simulink model "EMPlanner_cs2018"  (R2018a)
settings: Solver=ode5  StartTime=0.0  StopTime=120  FixedStep=1/1000  RelTol=1e-3
PreLoadFcn:
  | mbxruntime.callbacks.PreLoadFcn(bdroot);
PostLoadFcn:
  | mbxruntime.callbacks.PostLoadFcn(bdroot);
InitFcn:
  | mbxruntime.callbacks.InitFcn(bdroot);
StartFcn:
  | mbxruntime.callbacks.StartFcn(bdroot);
StopFcn:
  | mbxruntime.callbacks.StopFcn(bdroot);
model workspace (MAT data in the model file):
  mbox_table : struct (value not decoded)
  model_closed = 0
  sim_status = 0
undefined symbols (not defined in the file or in its folder): aubr, c_factor, cf, cr, DiscIntNeverNeededParam, global_path_x, global_path_y, KD_PID_distance, KD_PID_speed, KI_PID_distance, KI_PID_speed, KP_PID_distance, KP_PID_speed, la, lb, LQR_K1, LQR_K2, LQR_K3, LQR_K4, m, rack_displacement, right_wheel_ground, tablebr, vubr, vx_break_point, warningInitialVelocity, x0
libraries: PreScanSimulinkLibrary x21, simulink x19, simulink_extras x6, Solver_SF x1
(part 8 of 9)

== matlab function EMPlanner_cs2018/Audi_A8_Sedan_1/decision&planning module1/referenceline provider/MATLAB Function5 ==
  data: x_set input; match_point_index_set output; y_set input; frenet_path_x input; frenet_path_y input; frenet_path_heading input; frenet_path_kappa input; proj_x_set output; proj_y_set output; proj_heading_set output; proj_kappa_set output
function [match_point_index_set,proj_x_set,proj_y_set,proj_heading_set,proj_kappa_set] = ...
    fcn(x_set,y_set,frenet_path_x,frenet_path_y,frenet_path_heading,frenet_path_kappa)
%该函数将批量计算x_set，y_set中的xy，在frenet_path下的投影的信息
%输入 x_set,y_set，待投影的点的集合
%x_set,y_set,frenet_path_x,frenet_path_y,frenet_path_heading,frenet_path_kappa
%曲线在直角坐标系下的x，y，heading，kappa
%输出：match_point_index_set 匹配点在frenet_path下的编号的集合(即从全局路径第一个点开始数，第几个点是匹配点)
%     proj_x y heading kappa 投影的x,y,heading,kappa的集合

% 由于事先不知道x_set中到底有多少个点需要投影，因此事先声明一个最大的数量的点作为缓冲
n = 128;
% 并且由于不知道投影点的个数，所以也不知道输出的个数，因此输出也要做缓冲，用nan表示不存在的点
% 输出最多输出128个
% 输出初始化
match_point_index_set = ones(n,1) * nan;
proj_x_set = ones(n,1) * nan;
proj_y_set = ones(n,1) * nan;
proj_heading_set = ones(n,1) * nan;
proj_kappa_set = ones(n,1) * nan;

%找匹配点，需要利用上一个周期的结果作为下一个周期遍历的起点，因此需要声明两个全局变量
persistent is_first_run;
persistent pre_match_point_index_set;
persistent pre_frenet_path_x;
persistent pre_frenet_path_y;
persistent pre_frenet_path_heading;
persistent pre_frenet_path_kappa;
%算法主函数入口

if isempty(is_first_run)
    %该if分支表示函数首次运行
    is_first_run = 0;
    pre_frenet_path_x = frenet_path_x;
    pre_frenet_path_y = frenet_path_y;
    pre_frenet_path_heading = frenet_path_heading;
    pre_frenet_path_kappa = frenet_path_kappa;
    %要记录首次运行计算的匹配点的结果供下个周期运行，先初始化
    pre_match_point_index_set = ones(n,1) * nan;
    %对x_set,y_set的点做遍历，找到他们的匹配点
    for i = 1 : length(x_set)
        %首次运行时，没有任何提示，只能从frenet path的第一个点开始找
        if isnan(x_set(i))
            break;
        end
        start_search_index = 1;
        % 声明increase_count，用于表示在遍历时distance连续增加的个数
        increase_count = 0;
        % 开始遍历
        min_distance = inf;
        for j = start_search_index : length(frenet_path_x)
            distance = (x_set(i) - frenet_path_x(j))^2 + (y_set(i) - frenet_path_y(j))^2;
            if distance < min_distance
                min_distance = distance;
                match_point_index_set(i) = j;
                increase_count = 0;
            else
                increase_count = increase_count + 1;
            end
            %如果distance连续增加50次就不要再遍历了，节省时间
            if increase_count > 50
                break;
            end
        end
        
        %如何通过匹配点计算投影点，请参见《自动驾驶控制算法第七讲》
        %或《自动驾驶决策规划算法》第一章第三节
        
        %取出匹配点的编号
        match_point_index = match_point_index_set(i);
        %取出匹配点的信息
        match_point_x = frenet_path_x(match_point_index);
        match_point_y = frenet_path_y(match_point_index);
        match_point_heading = frenet_path_heading(match_point_index);
        match_point_kappa = frenet_path_kappa(match_point_index);
        %计算匹配点的方向向量与法向量
        vector_match_point = [match_point_x;match_point_y];
        vector_match_point_direction = [cos(match_point_heading);sin(match_point_heading)];
        %声明待投影点的位矢
        vector_r = [x_set(i);y_set(i)];
        
       %通过匹配点计算投影点
       vector_d = vector_r - vector_match_point;
       ds = vector_d' * vector_match_point_direction;
       vector_proj_point = vector_match_point + ds * vector_match_point_direction;
       proj_heading = match_point_heading + match_point_kappa * ds;
       proj_kappa = match_point_kappa;
       %计算结果输出
       proj_x_set(i) = vector_proj_point(1);
       proj_y_set(i) = vector_proj_point(2);
       proj_heading_set(i) = proj_heading;
       proj_kappa_set(i) = proj_kappa;
    end
    %匹配点的计算结果保存，供下一个周期使用
    pre_match_point_index_set = match_point_index_set;
else
    %此if分支表示不是首次运行
    
    %对每个x_set上的点做处理
    for i = 1 : length(x_set)
        %不是首次运行，对于点x_set(i),y_set(i)来说,start_search_index =
        %pre_match_point_index_set(i)
        start_search_index = pre_match_point_index_set(i);%上个周期匹配点的编号作为本周期搜索的起点
        %%%%%%%%%%%%
        increase_count_limit = 5;
        if isnan(start_search_index)
            increase_count_limit = 50;
            start_search_index = 1;
        end
        %%%%%%%%%%%%%%
        % 声明increase_count，用于表示在遍历时distance连续增加的个数
        increase_count = 0;
        % 开始遍历
        %这里多一个步骤，判断遍历的方向
        %计算上个周期匹配点的位矢
        vector_pre_match_point = [pre_frenet_path_x(start_search_index);pre_frenet_path_y(start_search_index)];
        vector_pre_match_point_direction = ...
            [cos(pre_frenet_path_heading(start_search_index));sin(pre_frenet_path_heading(start_search_index))];
        %判断遍历的方向
        flag = ([x_set(i);y_set(i)] - vector_pre_match_point)' * vector_pre_match_point_direction;
        min_distance = inf;
        if flag > 0.001
            for j = start_search_index : length(frenet_path_x)
                distance = (x_set(i) - frenet_path_x(j))^2 + (y_set(i) - frenet_path_y(j))^2;
                if distance < min_distance
                    min_distance = distance;
                    match_point_index_set(i) = j;
                    increase_count = 0;
                else
                    increase_count = increase_count + 1;
                end
                %如果distance连续增加5次就不要再遍历了，节省时间
                if increase_count > 5
                    break;
                end
            end
        elseif flag < - 0.001
            for j = start_search_index : -1 : 1
                distance = (x_set(i) - frenet_path_x(j))^2 + (y_set(i) - frenet_path_y(j))^2;
                if distance < min_distance
                    min_distance = distance;
                    match_point_index_set(i) = j;
                    increase_count = 0;
                else
                    increase_count = increase_count + 1;
                end
                %如果distance连续增加5次就不要再遍历了，节省时间
                if increase_count > increase_count_limit
                    break;
                end
            end
        else
            match_point_index_set(i) = start_search_index;
        end
        
        %如何通过匹配点计算投影点，请参见《自动驾驶控制算法第七讲》
        %或《自动驾驶决策规划算法》第一章第三节
        
        %取出匹配点的编号
        match_point_index = match_point_index_set(i);
        %取出匹配点的信息
        match_point_x = frenet_path_x(match_point_index);
        match_point_y = frenet_path_y(match_point_index);
        match_point_heading = frenet_path_heading(match_point_index);
        match_point_kappa = frenet_path_kappa(match_point_index);
        %计算匹配点的方向向量与法向量
        vector_match_point = [match_point_x;match_point_y];
        vector_match_point_direction = [cos(match_point_heading);sin(match_point_heading)];
        %声明待投影点的位矢
        vector_r = [x_set(i);y_set(i)];
        
       %通过匹配点计算投影点
       vector_d = vector_r - vector_match_point;
       ds = vector_d' * vector_match_point_direction;
       vector_proj_point = vector_match_point + ds * vector_match_point_direction;
       proj_heading = match_point_heading + match_point_kappa * ds;
       proj_kappa = match_point_kappa;
       %计算结果输出
       proj_x_set(i) = vector_proj_point(1);
       proj_y_set(i) = vector_proj_point(2);
       proj_heading_set(i) = proj_heading;
       proj_kappa_set(i) = proj_kappa;
  
    end
    %匹配点的计算结果保存，供下一个周期使用
    pre_match_point_index_set = match_point_index_set;
    pre_frenet_path_x = frenet_path_x;
    pre_frenet_path_y = frenet_path_y;
    pre_frenet_path_heading = frenet_path_heading;
    pre_frenet_path_kappa = frenet_path_kappa;
end

== matlab function EMPlanner_cs2018/Audi_A8_Sedan_1/perception module/data handle and transfer ==
  data: range input; obs_x_set_global output; theta input; velocity input; velocity_heading input; host_x input; host_y input; host_heading input; obs_y_set_global output; obs_velocity_set_global output; obs_heading_set_global output
function [obs_x_set_global,obs_y_set_global,obs_velocity_set_global,obs_heading_set_global] = fcn(range,theta,velocity,velocity_heading,host_x,host_y,host_heading)
%%%数据处理与坐标转换
obs_x_set_global = ones(32,1) * nan ;
obs_y_set_global = ones(32,1) * nan;
obs_velocity_set_global = ones(32,1) * nan;
obs_heading_set_global = ones(32,1) * nan;
theta_transfer = -1 * theta * pi / 180;
heading_transfer = (-velocity_heading + ones(32,1)*90) * pi / 180 ;
x_transfer = range .* cos(theta_transfer + host_heading);
y_transfer = range .* sin(theta_transfer + host_heading);
for i = 1:32
    if range(i) ~= 0
        obs_x_set_global(i) = x_transfer(i) + host_x + 2.16*cos(host_heading);
        obs_y_set_global(i) = y_transfer(i) + host_y + 2.16*sin(host_heading);
        obs_heading_set_global(i) = heading_transfer(i);
        obs_velocity_set_global(i) = velocity(i);
    end
end

== matlab function EMPlanner_cs2018/Audi_A8_Sedan_2/PathFollower_Preview_1/LateralController/Calculate delta steering error/eml_delta_steering_error ==
  data: v_x_vehicle input; v_x_vehicle_Min input; t_Preview_LatCtrl input; delta_steeringwheeltotal output; v_y_vehicle input; yawrate_vehicle input; CorneringStiffness_Tyres_Front input; CorneringStiffness_Tyres_Rear input; m_vehicle_total input; inertia_z_vehicle_total input; e_Lat input size=10; Pos_x_CoG_Vehicle input; wheelbase input; RefreshCounter parameter
function delta_steeringwheeltotal = eml_delta_steering_error(v_x_vehicle,v_x_vehicle_Min,t_Preview_LatCtrl,v_y_vehicle,yawrate_vehicle,CorneringStiffness_Tyres_Front,CorneringStiffness_Tyres_Rear,m_vehicle_total,inertia_z_vehicle_total,e_Lat,Pos_x_CoG_Vehicle,wheelbase,RefreshCounter)

delta_steeringwheeltotal = emlfcn_delta_steering_error(v_x_vehicle,v_x_vehicle_Min,t_Preview_LatCtrl,v_y_vehicle,yawrate_vehicle,CorneringStiffness_Tyres_Front,CorneringStiffness_Tyres_Rear,m_vehicle_total,inertia_z_vehicle_total,e_Lat,Pos_x_CoG_Vehicle,wheelbase,RefreshCounter);

% end function

== matlab function EMPlanner_cs2018/Audi_A8_Sedan_1/decision&planning module1/EM Planner/MATLAB Function7 ==
  data: s input; trajectory_x output; s_dot input; s_dot2 input; relative_time input; current_time input; path_s input; trajectory_x_init input; trajectory_y_init input; trajectory_heading_init input; trajectory_kappa_init input; trajectory_y output; trajectory_heading output; trajectory_kappa output; trajectory_speed output; trajectory_accel output; trajectory_time output
function [trajectory_x,trajectory_y,trajectory_heading,trajectory_kappa,trajectory_speed,trajectory_accel,trajectory_time] = ...
    fcn(s,s_dot,s_dot2,relative_time,current_time,path_s,trajectory_x_init,trajectory_y_init,trajectory_heading_init,trajectory_kappa_init)

n = 401;
trajectory_x = zeros(n,1);
trajectory_y = zeros(n,1);
trajectory_heading = zeros(n,1);
trajectory_kappa = zeros(n,1);
trajectory_speed = zeros(n,1);

trajectory_accel = zeros(n,1);

trajectory_time = zeros(n,1);
for i = 1:n-1
    trajectory_x(i) = interp1(path_s,trajectory_x_init,s(i));
    trajectory_y(i) = interp1(path_s,trajectory_y_init,s(i));
    trajectory_heading(i) = interp1(path_s,trajectory_heading_init,s(i));
    trajectory_kappa(i) = interp1(path_s,trajectory_kappa_init,s(i));
    trajectory_time(i) = relative_time(i) + current_time;
    trajectory_speed(i) = s_dot(i);
    trajectory_accel(i) = s_dot2(i);
end
trajectory_x(end) = trajectory_x_init(end);
trajectory_y(end) = trajectory_y_init(end);
trajectory_heading(end) = trajectory_heading_init(end);
trajectory_kappa(end) = trajectory_kappa_init(end);
trajectory_time(end) = relative_time(end) + current_time;
trajectory_speed(end) = s_dot(end);
trajectory_accel(end) = s_dot2(end);

== matlab function EMPlanner_cs2018/Audi_A8_Sedan_1/decision&planning module1/EM Planner/path decision and planning/generate obs SL/MATLAB Function5 ==
  data: x_set input; match_point_index_set output; y_set input; frenet_path_x input; frenet_path_y input; frenet_path_heading input; frenet_path_kappa input; proj_x_set output; proj_y_set output; proj_heading_set output; proj_kappa_set output
function [match_point_index_set,proj_x_set,proj_y_set,proj_heading_set,proj_kappa_set] = ...
    fcn(x_set,y_set,frenet_path_x,frenet_path_y,frenet_path_heading,frenet_path_kappa)
%该函数将批量计算x_set，y_set中的xy，在frenet_path下的投影的信息
%输入 x_set,y_set，待投影的点的集合
%x_set,y_set,frenet_path_x,frenet_path_y,frenet_path_heading,frenet_path_kappa
%曲线在直角坐标系下的x，y，heading，kappa
%输出：match_point_index_set 匹配点在frenet_path下的编号的集合(即从全局路径第一个点开始数，第几个点是匹配点)
%     proj_x y heading kappa 投影的x,y,heading,kappa的集合

% 由于事先不知道x_set中到底有多少个点需要投影，因此事先声明一个最大的数量的点作为缓冲
n = 128;
% 并且由于不知道投影点的个数，所以也不知道输出的个数，因此输出也要做缓冲，用nan表示不存在的点
% 输出最多输出128个
% 输出初始化
match_point_index_set = ones(n,1) * nan;
proj_x_set = ones(n,1) * nan;
proj_y_set = ones(n,1) * nan;
proj_heading_set = ones(n,1) * nan;
proj_kappa_set = ones(n,1) * nan;

%找匹配点，需要利用上一个周期的结果作为下一个周期遍历的起点，因此需要声明两个全局变量
persistent is_first_run;
persistent pre_match_point_index_set;
persistent pre_frenet_path_x;
persistent pre_frenet_path_y;
persistent pre_frenet_path_heading;
persistent pre_frenet_path_kappa;
%算法主函数入口

if isempty(is_first_run)
    %该if分支表示函数首次运行
    is_first_run = 0;
    pre_frenet_path_x = frenet_path_x;
    pre_frenet_path_y = frenet_path_y;
    pre_frenet_path_heading = frenet_path_heading;
    pre_frenet_path_kappa = frenet_path_kappa;
    %要记录首次运行计算的匹配点的结果供下个周期运行，先初始化
    pre_match_point_index_set = ones(n,1) * nan;
    %对x_set,y_set的点做遍历，找到他们的匹配点
    for i = 1 : length(x_set)
        if isnan(x_set(i))
            break;
        end
        %首次运行时，没有任何提示，只能从frenet path的第一个点开始找
        start_search_index = 1;
        % 声明increase_count，用于表示在遍历时distance连续增加的个数
        increase_count = 0;
        % 开始遍历
        min_distance = inf;
        for j = start_search_index : length(frenet_path_x)
            distance = (x_set(i) - frenet_path_x(j))^2 + (y_set(i) - frenet_path_y(j))^2;
            if distance < min_distance
                min_distance = distance;
                match_point_index_set(i) = j;
                increase_count = 0;
            else
                increase_count = increase_count + 1;
            end
            %如果distance连续增加50次就不要再遍历了，节省时间
            if increase_count > 50
                break;
            end
        end
        
        %如何通过匹配点计算投影点，请参见《自动驾驶控制算法第七讲》
        %或《自动驾驶决策规划算法》第一章第三节
        
        %取出匹配点的编号
        match_point_index = match_point_index_set(i);
        %取出匹配点的信息
        match_point_x = frenet_path_x(match_point_index);
        match_point_y = frenet_path_y(match_point_index);
        match_point_heading = frenet_path_heading(match_point_index);
        match_point_kappa = frenet_path_kappa(match_point_index);
        %计算匹配点的方向向量与法向量
        vector_match_point = [match_point_x;match_point_y];
        vector_match_point_direction = [cos(match_point_heading);sin(match_point_heading)];
        %声明待投影点的位矢
        vector_r = [x_set(i);y_set(i)];
        
       %通过匹配点计算投影点
       vector_d = vector_r - vector_match_point;
       ds = vector_d' * vector_match_point_direction;
       vector_proj_point = vector_match_point + ds * vector_match_point_direction;
       proj_heading = match_point_heading + match_point_kappa * ds;
       proj_kappa = match_point_kappa;
       %计算结果输出
       proj_x_set(i) = vector_proj_point(1);
       proj_y_set(i) = vector_proj_point(2);
       proj_heading_set(i) = proj_heading;
       proj_kappa_set(i) = proj_kappa;
    end
    %匹配点的计算结果保存，供下一个周期使用
    pre_match_point_index_set = match_point_index_set;
else
    %此if分支表示不是首次运行
    
    %对每个x_set上的点做处理
    for i = 1 : length(x_set)
        %不是首次运行，对于点x_set(i),y_set(i)来说,start_search_index =
        %pre_match_point_index_set(i)
        start_search_index = pre_match_point_index_set(i);%上个周期匹配点的编号作为本周期搜索的起点
        %%%%%%%%%%%%
        increase_count_limit = 5;
        if isnan(start_search_index)
            increase_count_limit = 50;
            start_search_index = 1;
        end
        %%%%%%%%%%%%%%
        % 声明increase_count，用于表示在遍历时distance连续增加的个数
        increase_count = 0;
        % 开始遍历
        %这里多一个步骤，判断遍历的方向
        %计算上个周期匹配点的位矢
        vector_pre_match_point = [pre_frenet_path_x(start_search_index);pre_frenet_path_y(start_search_index)];
        vector_pre_match_point_direction = ...
            [cos(pre_frenet_path_heading(start_search_index));sin(pre_frenet_path_heading(start_search_index))];
        %判断遍历的方向
        flag = ([x_set(i);y_set(i)] - vector_pre_match_point)' * vector_pre_match_point_direction;
        min_distance = inf;
        if flag > 0.001
            for j = start_search_index : length(frenet_path_x)
                distance = (x_set(i) - frenet_path_x(j))^2 + (y_set(i) - frenet_path_y(j))^2;
                if distance < min_distance
                    min_distance = distance;
                    match_point_index_set(i) = j;
                    increase_count = 0;
                else
                    increase_count = increase_count + 1;
                end
                %如果distance连续增加5次就不要再遍历了，节省时间
                if increase_count > 5
                    break;
                end
            end
        elseif flag < - 0.001
            for j = start_search_index : -1 : 1
                distance = (x_set(i) - frenet_path_x(j))^2 + (y_set(i) - frenet_path_y(j))^2;
                if distance < min_distance
                    min_distance = distance;
                    match_point_index_set(i) = j;
                    increase_count = 0;
                else
                    increase_count = increase_count + 1;
                end
                %如果distance连续增加5次就不要再遍历了，节省时间
                if increase_count > increase_count_limit
                    break;
                end
            end
        else
            match_point_index_set(i) = start_search_index;
        end
        
        %如何通过匹配点计算投影点，请参见《自动驾驶控制算法第七讲》
        %或《自动驾驶决策规划算法》第一章第三节
        
        %取出匹配点的编号
        match_point_index = match_point_index_set(i);
        %取出匹配点的信息
        match_point_x = frenet_path_x(match_point_index);
        match_point_y = frenet_path_y(match_point_index);
        match_point_heading = frenet_path_heading(match_point_index);
        match_point_kappa = frenet_path_kappa(match_point_index);
        %计算匹配点的方向向量与法向量
        vector_match_point = [match_point_x;match_point_y];
        vector_match_point_direction = [cos(match_point_heading);sin(match_point_heading)];
        %声明待投影点的位矢
        vector_r = [x_set(i);y_set(i)];
        
       %通过匹配点计算投影点
       vector_d = vector_r - vector_match_point;
       ds = vector_d' * vector_match_point_direction;
       vector_proj_point = vector_match_point + ds * vector_match_point_direction;
       proj_heading = match_point_heading + match_point_kappa * ds;
       proj_kappa = match_point_kappa;
       %计算结果输出
       proj_x_set(i) = vector_proj_point(1);
       proj_y_set(i) = vector_proj_point(2);
       proj_heading_set(i) = proj_heading;
       proj_kappa_set(i) = proj_kappa;
  
    end
    %匹配点的计算结果保存，供下一个周期使用
    pre_match_point_index_set = match_point_index_set;
    pre_frenet_path_x = frenet_path_x;
    pre_frenet_path_y = frenet_path_y;
    pre_frenet_path_heading = frenet_path_heading;
    pre_frenet_path_kappa = frenet_path_kappa;
end

== stateflow chart EMPlanner_cs2018/Audi_A8_Sedan_1/Chart ==
  (default) -> (junction 5)
  (junction 5) -> (junction 7)
  (junction 7) -> (junction 9) [order 1] : [i >= 100]
  (junction 7) -> (junction 13) [order 2] : {
      | i = i + 1;
      | }
  (junction 9) -> (junction 11) : {
      | do_planning;
      | i = 1;
      | }
  (junction 11) -> (junction 13)
  (junction 13) -> (junction 16)
  (junction 16) -> (junction 18) [order 1] : [j >= 10]
  (junction 16) -> (junction 22) [order 2] : {
      | j = j + 1;
      | }
  (junction 18) -> (junction 20) : {
      | do_control;
      | j = 1;
      | }
  (junction 20) -> (junction 22)
  (junction 22) -> (junction 25)
  data: i local =1; j local =1; k local =1
  events: do_planning output FUNCTION_CALL_EVENT; do_control output FUNCTION_CALL_EVENT

== matlab function EMPlanner_cs2018/Audi_A8_Sedan_1/decision&planning module1/EM Planner/MATLAB Function1 ==
  data: qp_path_s input; qp_path_l input; dp_path_s input; dp_path_l input; l_lb input; l_ub input
function  fcn(qp_path_s,qp_path_l,dp_path_s,dp_path_l,l_lb,l_ub)
coder.extrinsic('plot')
plot(qp_path_s,qp_path_l,dp_path_s,dp_path_l,dp_path_s,l_lb,dp_path_s,l_ub);

== matlab function EMPlanner_cs2018/Audi_A8_Sedan_1/decision&planning module1/EM Planner/MATLAB Function8 ==
  data: trajectory_x input; trajectory_x_final output; trajectory_y input; trajectory_heading input; trajectory_kappa input; trajectory_speed input; trajectory_accel input; trajectory_time input; stitch_x input; stitch_y input; stitch_heading input; stitch_kappa input; stitch_speed input; stitch_accel input; stitch_time input; trajectory_y_final output; trajectory_heading_final output; trajectory_kappa_final output; trajectory_speed_final output; trajectory_accel_final output; trajectory_time_final output
function [trajectory_x_final,trajectory_y_final,trajectory_heading_final,trajectory_kappa_final,...
          trajectory_speed_final,trajectory_accel_final,trajectory_time_final] = fcn(trajectory_x,...
          trajectory_y,trajectory_heading,trajectory_kappa,trajectory_speed,trajectory_accel,trajectory_time,...
          stitch_x,stitch_y,stitch_heading,stitch_kappa,stitch_speed,stitch_accel,stitch_time)
n = 401 + 20;
trajectory_x_final = zeros(n,1);
trajectory_y_final = zeros(n,1);
trajectory_heading_final = zeros(n,1);
trajectory_kappa_final = zeros(n,1);
trajectory_speed_final = zeros(n,1);
trajectory_accel_final = zeros(n,1);
trajectory_time_final = zeros(n,1);

trajectory_x_final = [stitch_x;trajectory_x];
trajectory_y_final = [stitch_y;trajectory_y];
trajectory_heading_final = [stitch_heading;trajectory_heading];
trajectory_kappa_final = [stitch_kappa;trajectory_kappa];
trajectory_speed_final = [stitch_speed;trajectory_speed];
trajectory_accel_final = [stitch_accel;trajectory_accel];
trajectory_time_final = [stitch_time;trajectory_time];

== matlab function EMPlanner_cs2018/Audi_A8_Sedan_1/control module1/control main/chassic steering system/MATLAB Function ==
  data: u input; right_steer output; la input; lb input
function right_steer = fcn(u,la,lb)
if abs(u)<1e-2
   right_steer = u;
else
   R =  (la+lb)/tan(u);
   right_steer = atan((la+lb)/(R+1.624/2));
end

== matlab function EMPlanner_cs2018/Audi_A8_Sedan_1/control module1/control main/lateral control LQR/calc lqr K ==
  data: k1 input; k output; k2 input; k3 input; k4 input; vx input
function k  = fcn(k1,k2,k3,k4,vx)
    if abs(vx)<0.1
        k=[0,0,0,0];
    else
       
        k=[k1,k2,k3,k4];
    end
end

== matlab function EMPlanner_cs2018/Audi_A8_Sedan_1/control module1/control main/lateral control LQR/err_kappa_calculate_module ==
  data: x input; y input; phi input; vx input; vy input; phi_dot input; xr input; yr input; thetar input; kappar input; err output; es output; s_dot output; phi output; projection_point_thetar output
function [err,es,s_dot,phi,projection_point_thetar] = fcn(x,y,phi,vx,vy,phi_dot,xr,yr,thetar,kappar)
    
    tor=[cos(thetar);sin(thetar)];
    nor=[-sin(thetar);cos(thetar)];
    d_err=[x-xr;y-yr];
    ed=nor'*d_err;
    es=tor'*d_err;
    %projection_point_thetar=thetar(dmin);%apollo
    projection_point_thetar=thetar+kappar*es;
    ed_dot=vy*cos(phi-projection_point_thetar)+vx*sin(phi-projection_point_thetar);
    %%%%%%%%%
    ephi=sin(phi-projection_point_thetar);
    %%%%%%%%%
    ss_dot=vx*cos(phi-projection_point_thetar)-vy*sin(phi-projection_point_thetar);
    s_dot=ss_dot/(1-kappar*ed);
    ephi_dot=phi_dot-kappar*s_dot;
    err=[ed;ed_dot;ephi;ephi_dot];
    
    
    
    
    
    
    
    
    
    
    
    


end

== matlab function EMPlanner_cs2018/Audi_A8_Sedan_1/control module1/control main/lateral control LQR/feed_forword_control ==
  data: vx input; a input; forword_angle output; b input; m input; cf input; cr input; k input; kr input
function forword_angle = fcn(vx,a,b,m,cf,cr,k,kr)
    forword_angle=kr*(a+b-b*k(3)-(m*vx*vx/(a+b))*((b/cf)+(a/cr)*k(3)-(a/cr)));
end

== matlab function EMPlanner_cs2018/Audi_A8_Sedan_1/control module1/control main/lateral control LQR/feedback_control+feedforword_control ==
  data: k input; angle output; err input; forword_angle input
function angle = fcn(k,err,forword_angle)

    angle=-k*err+forword_angle;
end

== matlab function EMPlanner_cs2018/Audi_A8_Sedan_1/control module1/control main/lateral control LQR/predict_module ==
  data: x input; pred_x_ctrl output; y input; phi input; vx input; vy input; phi_dot input; ts input; pred_y_ctrl output; pred_yaw_ctrl output; pred_vx_ctrl output; pred_vy_ctrl output; pred_yaw_dot_ctrl output
function [pred_x_ctrl,pred_y_ctrl,pred_yaw_ctrl,pred_vx_ctrl,pred_vy_ctrl,pred_yaw_dot_ctrl] = fcn(x,y,phi,vx,vy,phi_dot,ts)
    pred_x_ctrl=x+vx*ts*cos(phi)-vy*ts*sin(phi);
    pred_y_ctrl=y+vy*ts*cos(phi)+vx*ts*sin(phi);
    pred_yaw_ctrl=phi;
    pred_vx_ctrl=vx;
    pred_vy_ctrl=vy;
    pred_yaw_dot_ctrl=phi_dot;
end

== matlab function EMPlanner_cs2018/Audi_A8_Sedan_1/control module1/control main/longitudinal control double PID/MATLAB Function1 ==
  data: u input; throttle output; brake output
function [throttle,brake] = fcn(u)
    if u>=0
        throttle=u;
        brake=0;
    else
        throttle=0;
        brake=-u;
    end

== matlab function EMPlanner_cs2018/Audi_A8_Sedan_1/decision&planning module1/EM Planner/path decision and planning/MATLAB Function1 ==
  data: dp_path_s input; l_lb output; dp_path_l input; obs_s_set input; obs_l_set input; l_ub output
function [l_lb,l_ub] = fcn(dp_path_s,dp_path_l,obs_s_set,obs_l_set)
    l_lb = ones(120,1)*(-10);
    l_ub = ones(120,1)*10;
    %生成凸空间涉及区间合并
    %首先要计算到底有多少个静态障碍物
    for obs_count = 1:length(obs_s_set)
        if isnan(obs_s_set(obs_count))
            break;
        end
    end
    obs_count = obs_count - 1;
    if obs_count == 0
        return;
    end
    for i = 1:obs_count
        obs_s = obs_s_set(i);
        obs_l = obs_l_set(i);
        for j = 1:length(dp_path_s) - 1
            if dp_path_s(j) < obs_s && dp_path_s(j+1) > obs_s
                break;
            end
        end
        path_l = dp_path_l(j);
        if j <= 6
           interval_left_index = 1;
           interval_right_index = 10;
        elseif j >= length(dp_path_s) - 5
           interval_right_index = length(dp_path_s);
           interval_left_index = length(dp_path_s) - 9;
        else
           interval_left_index = j - 4;
           interval_right_index = j + 5;
        end
        for k = interval_left_index:interval_right_index
            if path_l >= obs_l
                l_lb_temp = obs_l + 2;
                if l_lb(k) < l_lb_temp
                    l_lb(k) = l_lb_temp;
                end
            else
                l_ub_temp = obs_l - 2;
                if l_ub(k) > l_ub_temp
                    l_ub(k) = l_ub_temp;
                end
            end       
        end      
    end
    
    
end

== matlab function EMPlanner_cs2018/Audi_A8_Sedan_1/decision&planning module1/EM Planner/MATLAB Function9 ==
  data: s_init input; s output; s_dot_init input; s_dot2_init input; relative_time_init input; s_dot output; s_dot2 output; relative_time output
function [s,s_dot,s_dot2,relative_time] = fcn(s_init,s_dot_init,s_dot2_init,relative_time_init)
%该函数将增密s s_dot s_dot2
T = relative_time_init(end);
n = 401;
dt = T/(n-1);
s = zeros(n,1);
s_dot = zeros(n,1);
s_dot2 = zeros(n,1);
relative_time = zeros(n,1);
for i = 1:n
    current_t = (i-1)*dt;
    for j = 1:length(relative_time_init)-1
        if relative_time_init(j) <= current_t && relative_time_init(j+1) > current_t
            break;
        end
    end
    x = current_t - relative_time_init(j);
    s(i) = s_init(j) + s_dot_init(j)*x + (1/3)*s_dot2_init(j)*x^2 + (1/6)*s_dot2_init(j+1)*x^2; 
    s_dot(i) = s_dot_init(j) + 0.5*s_dot2_init(j)*x + 0.5*s_dot2_init(j+1)*x;
    s_dot2(i) = s_dot2_init(j) + (s_dot2_init(j+1) - s_dot2_init(j))*x/(relative_time_init(j+1) - relative_time_init(j));
    relative_time(i) = current_t;
end

== matlab function EMPlanner_cs2018/Audi_A8_Sedan_1/decision&planning module1/EM Planner/path decision and planning/MATLAB Function2 ==
  data: dp_path_s input; l_lb input; l_ub input; path_start_l input; path_start_dl input; path_start_ddl input; w_cost_dl input; w_cost_ddl input; w_cost_dddl input; w_cost_ref input; qp_path_l output; qp_path_dl output; qp_path_ddl output
function [qp_path_l,qp_path_dl,qp_path_ddl]  = fcn(dp_path_s,l_lb,l_ub,path_start_l,path_start_dl,path_start_ddl,w_cost_dl,w_cost_ddl,w_cost_dddl,w_cost_ref)
qp_path_l = zeros(120,1);
qp_path_dl = zeros(120,1);
qp_path_ddl = zeros(120,1);
coder.extrinsic("quadprog")
%%%二次规划,三阶分段函数 l dl ddl
ds = dp_path_s(2) - dp_path_s(1);
% l(i+1) = l(i) + dl(i)*ds + (1/2)*ddl(i)*ds^2 + (1/6)*(dddl(i))*ds^3;
% dl(i+1) = dl(i) + ddl(i)*ds + (1/2)dddl(i)*ds^2   
%                                            [ 1
%                                              ds
%                                           (1/3)*ds^2
% [l(i) dl(i) ddl(i) l(i+1) dl(i+1) ddl(i+1)] -1
%                                              0
%                                           (1/6)*ds^2 
%                                              ]

%                                            [ 0
%                                              1
%                                            (1/2)*ds
% [l(i) dl(i) ddl(i) l(i+1) dl(i+1) ddl(i+1)]  0
%                                             -1   
%                                             ds/2
%                                              ] 
Aeq = zeros(3*120,2*120 - 2);
A1 = zeros(3*120,3*120);
A2 = zeros(3*120,3*120);
A3 = zeros(3*120,3*120);
A4 = zeros(3*120,120 - 1);
lb = ones(3*120,1)*-10;
ub = ones(3*120,1)*10;
beq = zeros(2*120 - 2,1);
f = zeros(3*120,1);
A_sub =[1,0;
        ds,1;
        (1/3)*ds^2,(1/2)*ds;
        -1,0;
        0,-1;
        (1/6)*ds^2,ds/2];
for i = 1:120 - 1
    Aeq(3*i-2:3*i+3,2*i-1:2*i) = A_sub;
end
for i = 1:120
    A1(3*i-2,3*i-2) = w_cost_ref;
    A2(3*i-1,3*i-1) = w_cost_dl;
    A3(3*i,3*i) = w_cost_ddl;
    lb(3*i-2) = l_lb(i);
    ub(3*i-2) = l_ub(i);
end
A4_sub =[0;0;1;0;0;-1];
for i = 1:120 - 1
   A4(3*i-2:3*i+3,i:i) = A4_sub;
end
lb(1) = path_start_l;
ub(1) = path_start_l;
lb(2) = path_start_dl;
ub(2) = path_start_dl;
lb(3) = path_start_ddl;
ub(3) = path_start_ddl;
H = A1 + A2 + A3 + w_cost_dddl*(A4*A4');
H = 2*H;
X = quadprog(H,f,[],[],Aeq',beq,lb,ub);
for i = 1:120
    qp_path_l(i) = X(3*i - 2);
    qp_path_dl(i) = X(3*i - 1);
    qp_path_ddl(i) = X(3*i);
end

== matlab function EMPlanner_cs2018/Audi_A8_Sedan_1/decision&planning module1/EM Planner/calc plan start gcs ==
  data: pre_trajectory_x input; plan_start_x output; pre_trajectory_y input; pre_trajectory_heading input; pre_trajectory_kappa input; pre_trajectory_velocity input; pre_trajectory_accel input; pre_trajectory_time_abs input; current_time input; host_x input; host_y input; host_heading_xy input; host_vx input; host_vy input; host_ax input; host_ay input; plan_start_y output; plan_start_heading output; plan_start_kappa output; plan_start_vx output; plan_start_vy output; plan_start_ax output; plan_start_ay output; plan_start_time output; stitch_x output; stitch_y output; stitch_heading output; stitch_kappa output; stitch_speed output; stitch_accel output; stitch_time output
function [plan_start_x,plan_start_y,plan_start_heading,plan_start_kappa,plan_start_vx,plan_start_vy,plan_start_ax,plan_start_ay,plan_start_time,...
    stitch_x,stitch_y,stitch_heading,stitch_kappa,stitch_speed,stitch_accel,stitch_time] = fcn(pre_trajectory_x,pre_trajectory_y,pre_trajectory_heading,pre_trajectory_kappa,pre_trajectory_velocity,pre_trajectory_accel,...
                 pre_trajectory_time_abs,current_time,host_x,host_y,host_heading_xy,host_vx,host_vy,host_ax,host_ay)
stitch_x = zeros(20,1);
stitch_y = zeros(20,1);
stitch_heading = zeros(20,1);
stitch_kappa = zeros(20,1);
stitch_speed = zeros(20,1);
stitch_accel = zeros(20,1);
temp = -20:1:-1;
stitch_time = temp';
persistent is_first_run;
if isempty(is_first_run)
    is_first_run = 0;
    plan_start_x = host_x;
    plan_start_y = host_y;
    plan_start_heading = host_heading_xy;
    plan_start_kappa = 0;
    plan_start_vx = host_vx*cos(host_heading_xy) - host_vy*sin(host_heading_xy);
    plan_start_vy = host_vx*sin(host_heading_xy) + host_vy*cos(host_heading_xy);
    plan_start_ax = host_ax*cos(host_heading_xy) - host_ay*sin(host_heading_xy);
    plan_start_ay = host_ax*sin(host_heading_xy) + host_ay*cos(host_heading_xy); 
    plan_start_time = current_time + 0.1;
else
    x_cur = host_x;
    y_cur = host_y;
    heading_cur = host_heading_xy;
    kappa_cur = 0;
    vx_cur = host_vx*cos(heading_cur) - host_vy*sin(heading_cur);
    vy_cur = host_vx*sin(heading_cur) + host_vy*cos(heading_cur);
    ax_cur = host_ax*cos(heading_cur) - host_ay*sin(heading_cur);
    ay_cur = host_ax*sin(heading_cur) + host_ay*cos(heading_cur);
    dt = 0.1;
    for k = 1:length(pre_trajectory_time_abs)
        if pre_trajectory_time_abs(k) ~= -1
            break;
        end
    end
    if current_time < pre_trajectory_time_abs(k)
        %当前时间比上一个轨迹的开头都要短
        plan_start_x = x_cur + vx_cur*dt +0.5*ax_cur * dt^2;
        plan_start_y = y_cur + vy_cur*dt + 0.5*ay_cur * dt^2;
        plan_start_vx = vx_cur + ax_cur * dt;
        plan_start_vy = vy_cur + ay_cur * dt;
        plan_start_heading = atan2(plan_start_vy,plan_start_vx);
        plan_start_ax = ax_cur;
        plan_start_ay = ay_cur;
        plan_start_kappa = kappa_cur;
        plan_start_time = current_time + 0.1;
        return;
    end
    for i = 1:length(pre_trajectory_time_abs)
        if (pre_trajectory_time_abs(i) <= current_time && pre_trajectory_time_abs(i+1) > current_time)
            break;
        end
    end
    pre_x_desire = pre_trajectory_x(i);
    pre_y_desire = pre_trajectory_y(i);
    pre_heading_desire = pre_trajectory_heading(i);
    d_err = [host_x;host_y] - [pre_x_desire;pre_y_desire];
    tor = [cos(pre_heading_desire);sin(pre_heading_desire)];
    nor = [-sin(pre_heading_desire);cos(pre_heading_desire)];
    lon_err = abs(d_err'*tor);
    lat_err = abs(d_err'*nor);
    if lon_err > 5 && lat_err > 5
        plan_start_x = x_cur + vx_cur*dt +0.5*ax_cur * dt^2;
        plan_start_y = y_cur + vy_cur*dt + 0.5*ay_cur * dt^2;
        plan_start_vx = vx_cur + ax_cur * dt;
        plan_start_vy = vy_cur + ay_cur * dt;
        plan_start_heading = atan2(plan_start_vy,plan_start_vx);
        plan_start_ax = ax_cur;
        plan_start_ay = ay_cur;
        plan_start_kappa = kappa_cur;
        plan_start_time = current_time + 0.1;
        return;
    else
        for j = i:length(pre_trajectory_time_abs)
            if (pre_trajectory_time_abs(j) <= current_time + 0.1 && pre_trajectory_time_abs(j+1) > current_time + 0.1)
                break;
            end
        end
        plan_start_x = pre_trajectory_x(j);
        plan_start_y = pre_trajectory_y(j);
        plan_start_heading = pre_trajectory_heading(j);
        plan_start_kappa = pre_trajectory_kappa(j);
        plan_start_vx = pre_trajectory_velocity(j)*cos(plan_start_heading);
        plan_start_vy = pre_trajectory_velocity(j)*sin(plan_start_heading);
        tor = [cos(plan_start_heading);sin(plan_start_heading)];
        nor = [-sin(plan_start_heading);cos(plan_start_heading)];
        a_tor = pre_trajectory_accel(j)*tor;
        a_nor = pre_trajectory_velocity(j)^2 * plan_start_kappa * nor;
        plan_start_ax = a_tor(1) + a_nor(1);
        plan_start_ay = a_tor(2) + a_nor(2);
        plan_start_time = pre_trajectory_time_abs(j);
        j = j - 1;
        if j >= 20
            stitch_x = pre_trajectory_x(j - 19:j);
            stitch_y = pre_trajectory_y(j - 19:j);
            stitch_heading = pre_trajectory_heading(j - 19:j);
            stitch_kappa = pre_trajectory_kappa(j - 19:j);
            stitch_speed = pre_trajectory_velocity(j - 19:j);
            stitch_accel = pre_trajectory_accel(j - 19:j);
            stitch_time = pre_trajectory_time_abs(j - 19:j);
        else
            stitch_x(20 - j +1:20) = pre_trajectory_x(1:j);
            stitch_y(20 - j +1:20) = pre_trajectory_y(1:j);
            stitch_heading(20 - j +1:20) = pre_trajectory_heading(1:j);
            stitch_kappa(20 - j +1:20) = pre_trajectory_kappa(1:j);
            stitch_speed(20 - j +1:20) = pre_trajectory_velocity(1:j);
            stitch_accel(20 - j +1:20) = pre_trajectory_velocity(1:j);
            stitch_time(20 - j +1:20) = pre_trajectory_time_abs(1:j);
        end
    end
end

== matlab function EMPlanner_cs2018/Audi_A8_Sedan_1/decision&planning module1/EM Planner/MATLAB Function3 ==
  data: s_set input; x_set output; l_set input; dl_set input; frenet_path_x input; frenet_path_y input; frenet_path_heading input; frenet_path_kappa input; index2s input; y_set output; theta_set output
function [x_set,y_set,theta_set] = fcn(s_set,l_set,dl_set,frenet_path_x,frenet_path_y,frenet_path_heading,frenet_path_kappa,index2s)
% 通用模块，从frenet到cartesian
n = 128;
x_set = ones(n,1)*nan;
y_set = ones(n,1)*nan;
theta_set = ones(n,1)*nan;
for i = 1:length(s_set)
    if isnan(s_set(i))
        break;
    end
    pre_index = -1;
    for j = 1:length(index2s)-1
        if (index2s(j) <= s_set(i)) && (index2s(j+1) > s_set(i))
            pre_index = j;
            break;
        end
    end
    if pre_index == -1
        return;
    end
    match_point_pre = [frenet_path_x(pre_index);frenet_path_y(pre_index)];
    ds = s_set(i) - index2s(pre_index);
    tor = [cos(frenet_path_heading(pre_index));sin(frenet_path_heading(pre_index))];
    nor = [-sin(frenet_path_heading(pre_index));cos(frenet_path_heading(pre_index))];
    proj_point = match_point_pre + ds*tor;
    proj_theta = frenet_path_heading(pre_index) + frenet_path_kappa(pre_index)*ds;
    real_point = proj_point + nor*l_set(i);
    x_set(i) = real_point(1);
    y_set(i) = real_point(2);
    theta_set(i) = proj_theta + atan(dl_set(i)/(1 - frenet_path_kappa(pre_index)*l_set(i)));
end

== matlab function EMPlanner_cs2018/Audi_A8_Sedan_1/decision&planning module1/EM Planner/General Cartesian2Frenet/MATLAB Function ==
  data: x_set input; y_set input; frenet_path_x input; s_set output; frenet_path_y input; proj_x_set input; proj_y_set input; proj_heading_set input; proj_match_point_index_set input; index2s input; l_set output
function [s_set,l_set] = fcn(x_set,y_set,frenet_path_x,frenet_path_y,proj_x_set,proj_y_set,proj_heading_set,proj_match_point_index_set,index2s)
    %该函数将计算x_set,y_set上的点在frenet_path上的sl
    %输入 x_set,y_set 待坐标转换的点
    %     frenet_path_x,frenet_path_y frenet坐标轴
    %     origin_x,origin_y 坐标原点
    %     origin_match_point_index 坐标原点的匹配点的编号
    %     proj_x_set,proj_y_set,proj_heading_set,proj_kappa_set,proj_match_point_index 待坐标转换的点的投影点的信息
    %     index2s index与弧长的转化表

    % 由于不知道有多少点需要做坐标转换，因此设置一个最大值作为缓冲
    n = 128; %最多处理128个点
    %输出初始化
    s_set = ones(n, 1)*nan;
    l_set = ones(n, 1)*nan;
    for i = 1:length(x_set)
        if isnan(x_set(i))
            break;
        end
        s_set(i) = CalcSFromIndex2S(index2s,frenet_path_x,frenet_path_y,proj_x_set(i),proj_y_set(i),proj_match_point_index_set(i));
        n_r = [-sin(proj_heading_set(i));cos(proj_heading_set(i))];
        r_h = [x_set(i);y_set(i)];
        r_r = [proj_x_set(i);proj_y_set(i)];
        l_set(i) = (r_h - r_r)' * n_r;
    end
end


function s = CalcSFromIndex2S(index2s,path_x,path_y,proj_x,proj_y,proj_match_point_index)
    %该函数将计算给定index2s的映射关系后，计算点(proj_x,proj_y)所对应的弧长
    %判断给定的坐标原点在匹配点的前面还是后面
    vector_1 = [proj_x;proj_y] - [path_x(proj_match_point_index);path_y(proj_match_point_index)];
    if (proj_match_point_index < length(path_x))
        vector_2 = [path_x(proj_match_point_index + 1);path_y(proj_match_point_index + 1)] - [path_x(proj_match_point_index);path_y(proj_match_point_index)];
    else
        vector_2 = [path_x(proj_match_point_index);path_y(proj_match_point_index)] - [path_x(proj_match_point_index - 1);path_y(proj_match_point_index - 1)];
    end
    if vector_1'*vector_2 > 0
        %坐标原点在匹配点前面
        s = index2s(proj_match_point_index) + sqrt(vector_1'*vector_1);
    else
        %坐标原点在匹配点后面
        s = index2s(proj_match_point_index) - sqrt(vector_1'*vector_1);
    end
end

== matlab function EMPlanner_cs2018/Audi_A8_Sedan_1/decision&planning module1/EM Planner/path decision and planning/MATLAB Function ==
  data: host_x input; obs_x_set_final output; host_y input; host_heading_xy input; obs_x_set_gcs input; obs_y_set_gcs input; obs_y_set_final output; obs_velocity_set_gcs input
function [obs_x_set_final,obs_y_set_final] = fcn(host_x,host_y,host_heading_xy,obs_x_set_gcs,obs_y_set_gcs,obs_velocity_set_gcs)
%初步筛选障碍物，只取纵向[-10,70] 横向[-10, 10]的障碍物的静态障碍物
n = 128;
obs_x_set_final = ones(n,1)*nan;
obs_y_set_final = ones(n,1)*nan;
count = 1;
for i = 1:length(obs_x_set_gcs)
    if isnan(obs_x_set_gcs(i))
        break;
    end
    if abs(obs_velocity_set_gcs(i)) > 0.1
        continue;
    end
    
    %车辆朝向切向量
    tor = [cos(host_heading_xy);sin(host_heading_xy)];
    nor = [-sin(host_heading_xy);cos(host_heading_xy)];
    %障碍物向量
    v_obs = [obs_x_set_gcs(i);obs_y_set_gcs(i)] - [host_x;host_y];
    %纵向距离
    lon_distance = v_obs'*tor;
    %横向距离
    lat_distance = v_obs'*nor;
    if (lon_distance < 70)&&(lon_distance > -10)&&(lat_distance < 10)&&(lat_distance > -10)
        obs_x_set_final(count) = obs_x_set_gcs(i);
        obs_y_set_final(count) = obs_y_set_gcs(i);
        count = count + 1;
    end
    
end

== matlab function EMPlanner_cs2018/Audi_A8_Sedan_1/control module1/MATLAB Function ==
  data: current_time input; xr_desire output; trajectory_x input; trajectory_y input; trajectory_heading input; trajectory_kappa input; trajectory_speed input; trajectory_accel input; trajectory_time input; yr_desire output; thetar_desire output; kappar_desire output; speed_desire output; accel_desire output
function [xr_desire,yr_desire,thetar_desire,kappar_desire,speed_desire,accel_desire] = fcn(current_time,trajectory_x,...
    trajectory_y,trajectory_heading,trajectory_kappa,trajectory_speed,trajectory_accel,trajectory_time)

for i = 1:length(trajectory_time)
    if trajectory_time(i) >= 0
        break;
    end
end

for j = 1:i
    trajectory_x(j) = trajectory_x(i);
    trajectory_y(j) = trajectory_y(i);
    trajectory_heading(j) = trajectory_heading(i);
    trajectory_kappa(j) = trajectory_kappa(i);
    trajectory_speed(j) = trajectory_speed(i);
    trajectory_accel(j) = trajectory_accel(i);
end
if trajectory_time(1) == 0
    xr_desire = 0;
    yr_desire = 0;
    thetar_desire = 0;
    kappar_desire = 0;
    speed_desire = 0;
    accel_desire = 0;
else
    xr_desire = spline(trajectory_time,trajectory_x,current_time);
    yr_desire = spline(trajectory_time,trajectory_y,current_time);
    thetar_desire = spline(trajectory_time,trajectory_heading,current_time);
    kappar_desire = spline(trajectory_time,trajectory_kappa,current_time);
    speed_desire = spline(trajectory_time,trajectory_speed,current_time);
    accel_desire = spline(trajectory_time,trajectory_accel,current_time);
end

== matlab function EMPlanner_cs2018/Audi_A8_Sedan_1/decision&planning module1/EM Planner/MATLAB Function5 ==
  data: trajectory_x input; path_s_end output; trajectory_y input; path_s output
function [path_s_end,path_s] = fcn(trajectory_x,trajectory_y)
n = length(trajectory_x);
path_s = zeros(n,1);
sum = 0;
for i = 2:length(trajectory_x)
    sum = sum + sqrt((trajectory_x(i) - trajectory_x(i-1))^2 + (trajectory_y(i) - trajectory_y(i-1))^2);
    path_s(i) = sum;
end
path_s_end = path_s(end);

== matlab function EMPlanner_cs2018/Audi_A8_Sedan_1/decision&planning module1/EM Planner/generate index to s ==
  data: path_x input; index2s output; path_y input; origin_x input; origin_y input; origin_match_point_index input
function index2s  = fcn(path_x,path_y,origin_x,origin_y,origin_match_point_index)
    %该算法将计算出index与s的转换关系，index2s(i)表示当编号为i时，对应的弧长s
    n = 181;
    index2s = zeros(n,1);
    %这个循环计算的是以轨迹起点为坐标原点的index2s的转换关系
    for i = 2:181
        index2s(i) = sqrt((path_x(i) - path_x(i-1))^2 + (path_y(i) - path_y(i-1))^2) + index2s(i-1);  
    end
    %再计算起点到坐标原点的弧长s0 ，减去s0,就得到了以给定的坐标原点为起点的index2s的关系
    s0 = CalcSFromIndex2S(index2s,path_x,path_y,origin_x,origin_y,origin_match_point_index);
    index2s = index2s - ones(n,1)*s0;
end

function s = CalcSFromIndex2S(index2s,path_x,path_y,proj_x,proj_y,proj_match_point_index)
    %该函数将计算给定index2s的映射关系后，计算点(proj_x,proj_y)所对应的弧长
    %判断给定的坐标原点在匹配点的前面还是后面
    vector_1 = [proj_x;proj_y] - [path_x(proj_match_point_index);path_y(proj_match_point_index)];
    if (proj_match_point_index < length(path_x))
        vector_2 = [path_x(proj_match_point_index + 1);path_y(proj_match_point_index + 1)] - [path_x(proj_match_point_index);path_y(proj_match_point_index)];
    else
        vector_2 = [path_x(proj_match_point_index);path_y(proj_match_point_index)] - [path_x(proj_match_point_index - 1);path_y(proj_match_point_index - 1)];
    end
    if vector_1'*vector_2 > 0
        %坐标原点在匹配点前面
        s = index2s(proj_match_point_index) + sqrt(vector_1'*vector_1);
    else
        %坐标原点在匹配点后面
        s = index2s(proj_match_point_index) - sqrt(vector_1'*vector_1);
    end
end
